simulink model "lct_simulation"  (R2023b)
settings: Solver=ode4  StartTime=0.0  StopTime=10.0  FixedStep=0.01  RelTol=1e-3
settings Model: Creator=charu  LastModifiedBy=charu

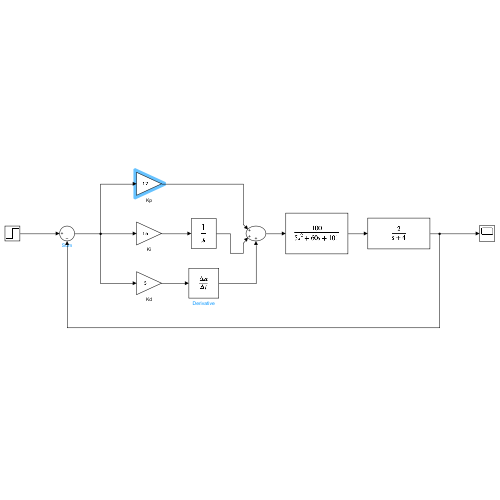
[thumbnail: Simulink's stored preview of the top-level diagram]
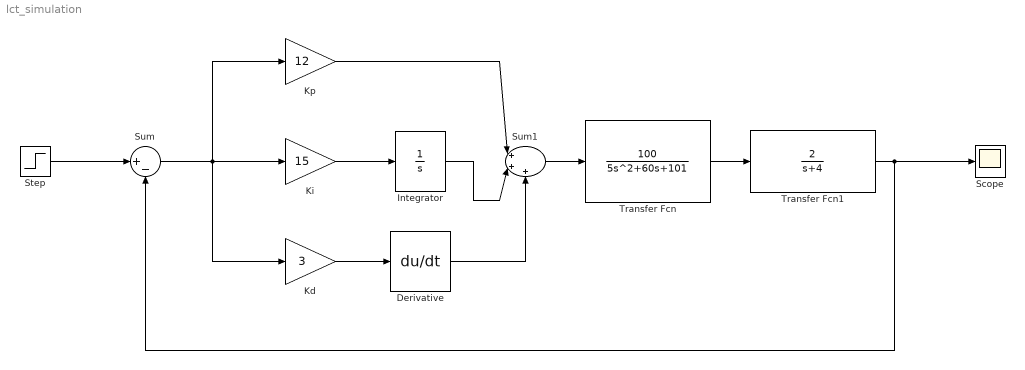
== system lct_simulation ==
  Derivative : Derivative
  Integrator : Integrator
  Kd : Gain  Gain=3
  Ki : Gain  Gain=15
  Kp : Gain  Gain=12
  Scope : Scope
  Step : Step  Time=0  SampleTime=0
  Sum : Sum  Inputs=|+-
  Sum1 : Sum  Inputs=|+++
  Transfer Fcn : TransferFcn  Numerator=[100]  Denominator=[5 60 101]
  Transfer Fcn1 : TransferFcn  Numerator=[2]  Denominator=[1 4]
  wires:
  Step/1 -> Sum/1
  Transfer Fcn1/1 -> Sum/2, Scope/1
  Transfer Fcn/1 -> Transfer Fcn1/1
  Sum/1 -> Kd/1, Ki/1, Kp/1
  Kd/1 -> Derivative/1
  Ki/1 -> Integrator/1
  Derivative/1 -> Sum1/3
  Integrator/1 -> Sum1/2
  Kp/1 -> Sum1/1
  Sum1/1 -> Transfer Fcn/1
